simulink subsystem "systemConfig"  (R2021a)
settings: Solver=VariableStepAuto  StartTime=0.0  StopTime=10.0  RelTol=1e-3
libraries: attitude_library x4
settings Model: Creator=Laura  LastModifiedBy=Laura

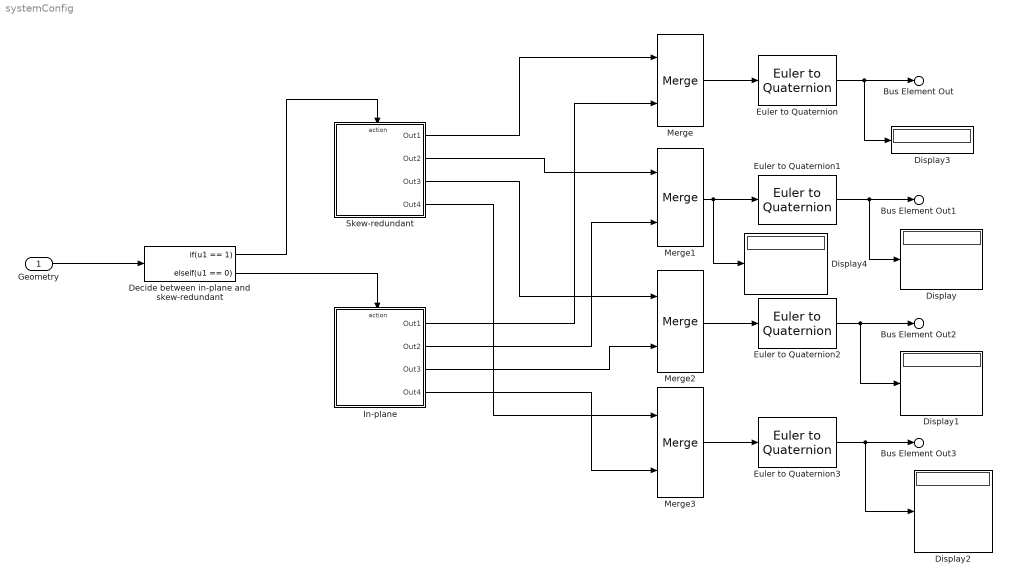
== system systemConfig ==
  Geometry : Inport
  Decide between in-plane and skew-redundant : If  IfExpression=u1 == 1  ElseIfExpressions=u1 == 0  ShowElse=off
  Display{,1..4} (5 alike) : Display
  Euler to Quaternion{,1..3} (4 alike) : attitude_library/Euler to Quaternion  SystemSampleTime=-1  VariantActivationTime=update diagram  Latency=0  AutoFrameSizeCalculation=off
      settings: SourceProductName=Attitude library
  In-plane : Subsystem  TreatAsAtomicUnit=on
  Merge{,1..3} (4 alike) : Merge
  Skew-redundant : Subsystem  TreatAsAtomicUnit=on
  Bus Element Out : Outport  PortName=CONFIG  Element=quat1_VB
  Bus Element Out1 : Outport  PortName=CONFIG  Element=quat2_VB
  Bus Element Out2 : Outport  PortName=CONFIG  Element=quat3_VB
  Bus Element Out3 : Outport  PortName=CONFIG  Element=quat4_VB
  wires:
  Euler to Quaternion3/1 -> Bus Element Out3/1, Display2/1
  In-plane/1(Out1) -> Merge/2
  In-plane/4(Out4) -> Merge3/2
  Skew-redundant/3(Out3) -> Merge2/1
  Decide between in-plane and skew-redundant/1 -> Skew-redundant/Action
  In-plane/2(Out2) -> Merge1/2
  Skew-redundant/4(Out4) -> Merge3/1
  Decide between in-plane and skew-redundant/2 -> In-plane/Action
  Merge/1 -> Euler to Quaternion/1
  Merge3/1 -> Euler to Quaternion3/1
  Merge1/1 -> Euler to Quaternion1/1, Display4/1
  Euler to Quaternion/1 -> Bus Element Out/1, Display3/1
  Merge2/1 -> Euler to Quaternion2/1
  In-plane/3(Out3) -> Merge2/2
  Skew-redundant/2(Out2) -> Merge1/1
  Euler to Quaternion2/1 -> Bus Element Out2/1, Display1/1
  Euler to Quaternion1/1 -> Bus Element Out1/1, Display/1
  Geometry/1 -> Decide between in-plane and skew-redundant/1
  Skew-redundant/1(Out1) -> Merge/1

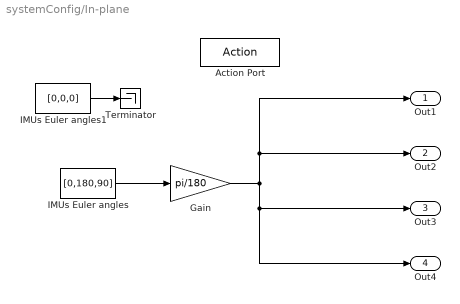
== system systemConfig/In-plane ==
  Action Port : ActionPort
  Gain : Gain  Gain=pi/180
  IMUs Euler angles : Constant  Value=[0,180,90]
  IMUs Euler angles1 : Constant  Value=[0,0,0]
  Terminator : Terminator
  Out1 : Outport
  Out2 : Outport  Port=2
  Out3 : Outport  Port=3
  Out4 : Outport  Port=4
  wires:
  IMUs Euler angles1/1 -> Terminator/1
  IMUs Euler angles/1 -> Gain/1
  Gain/1 -> Out3/1, Out4/1, Out2/1, Out1/1

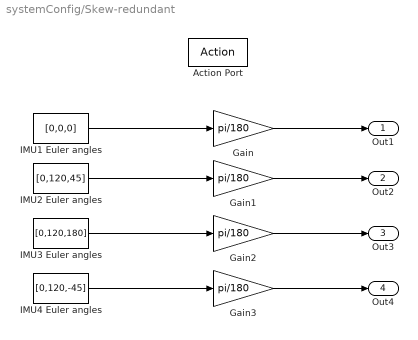
== system systemConfig/Skew-redundant ==
  Action Port : ActionPort
  Gain{,1..3} (4 alike) : Gain  Gain=pi/180
  IMU1 Euler angles : Constant  Value=[0,0,0]
  IMU2 Euler angles : Constant  Value=[0,120,45]
  IMU3 Euler angles : Constant  Value=[0,120,180]
  IMU4 Euler angles : Constant  Value=[0,120,-45]
  Out1 : Outport
  Out2 : Outport  Port=2
  Out3 : Outport  Port=3
  Out4 : Outport  Port=4
  wires:
  IMU1 Euler angles/1 -> Gain/1
  IMU2 Euler angles/1 -> Gain1/1
  IMU3 Euler angles/1 -> Gain2/1
  IMU4 Euler angles/1 -> Gain3/1
  Gain/1 -> Out1/1
  Gain1/1 -> Out2/1
  Gain2/1 -> Out3/1
  Gain3/1 -> Out4/1
